simulink model "paralell_robot_D_2021"  (R2021a)
settings: Solver=VariableStepAuto  StartTime=0.0  StopTime=4*1.2  RelTol=1e-3
values from neighbouring files (symbols this model uses):
  B = 1.0    (= 1)    [paralell_robot_parameters.m]    (also in trajectory_generation.m = zeros(18,1))
  g = 9.81    [paralell_robot_parameters.m]    (also in robot_param.m)
  G = 0.8    [paralell_robot_parameters.m]
  I1_x = 50    [paralell_robot_parameters.m]    (also in robot_param.m)
  I1_y = 50    [paralell_robot_parameters.m]    (also in robot_param.m)
  I1_z = 50    [paralell_robot_parameters.m]    (also in robot_param.m)
  I2_x = 1    [paralell_robot_parameters.m]    (also in robot_param.m)
  I2_y = 20    [paralell_robot_parameters.m]    (also in robot_param.m)
  I2_z = 20    [paralell_robot_parameters.m]    (also in robot_param.m)
  I3_x = 0.5    [paralell_robot_parameters.m]    (also in robot_param.m)
  I3_y = 8    [paralell_robot_parameters.m]    (also in robot_param.m)
  I3_z = 8    [paralell_robot_parameters.m]    (also in robot_param.m)
  I4_x = 10    [paralell_robot_parameters.m]    (also in robot_param.m = 1)
  I4_y = 10    [paralell_robot_parameters.m]    (also in robot_param.m)
  I4_z = 10    [paralell_robot_parameters.m]    (also in robot_param.m)
  I5_x = 0.2    [paralell_robot_parameters.m]    (also in robot_param.m)
  I5_y = 1    [paralell_robot_parameters.m]    (also in robot_param.m)
  I5_z = 1    [paralell_robot_parameters.m]    (also in robot_param.m)
  I6_x = 2    [paralell_robot_parameters.m]    (also in robot_param.m)
  I6_y = 3    [paralell_robot_parameters.m]    (also in robot_param.m)
  I6_z = 2    [paralell_robot_parameters.m]    (also in robot_param.m)
  I7_x = 1    [paralell_robot_parameters.m]    (also in robot_param.m)
  I7_y = 18    [paralell_robot_parameters.m]    (also in robot_param.m)
  I7_z = 18    [paralell_robot_parameters.m]    (also in robot_param.m)
  I8_x = 0.5    [paralell_robot_parameters.m]    (also in robot_param.m = 0.2)
  I8_y = 2    [paralell_robot_parameters.m]    (also in robot_param.m)
  I8_z = 2    [paralell_robot_parameters.m]    (also in robot_param.m)
  I9_x = 1    [paralell_robot_parameters.m]    (also in robot_param.m)
  I9_y = 1    [paralell_robot_parameters.m]    (also in robot_param.m)
  I9_z = 1    [paralell_robot_parameters.m]    (also in robot_param.m)
  L1 = 0.240    (= 0.24)    [paralell_robot_parameters.m]    (also in robot_param.m)
  L2 = 0.800    (= 0.8)    [paralell_robot_parameters.m]    (also in robot_param.m)
  L3 = 1.050    (= 1.05)    [paralell_robot_parameters.m]    (also in robot_param.m)
  L4 = 1.175    [paralell_robot_parameters.m]    (also in robot_param.m)
  L5 = 0.225    [paralell_robot_parameters.m]    (also in robot_param.m)
  L6 = 0.200    (= 0.2)    [paralell_robot_parameters.m]    (also in robot_param.m)
  L7 = 0.235    [paralell_robot_parameters.m]    (also in robot_param.m)
  L8 = 0.248    [paralell_robot_parameters.m]    (also in robot_param.m)
  m1 = 750    [paralell_robot_parameters.m]    (also in robot_param.m)
  m2 = 250    [paralell_robot_parameters.m]    (also in robot_param.m)
  m3 = 150    [paralell_robot_parameters.m]    (also in robot_param.m)
  m4 = 500    [paralell_robot_parameters.m]    (also in robot_param.m)
  m5 = 50    [paralell_robot_parameters.m]    (also in robot_param.m = 150)
  m6 = 150    [paralell_robot_parameters.m]
  m7 = 200    [paralell_robot_parameters.m]    (also in robot_param.m)
  m8 = 100    [paralell_robot_parameters.m]    (also in robot_param.m)
  m9 = 50    [paralell_robot_parameters.m]    (also in robot_param.m)
  N = length(pt)-1    [trajectory_generation_quintic.m]
  PB = T+0.02    (= 0.12)    [paralell_robot_parameters.m]
  R = 0.0    (= 0)    [paralell_robot_parameters.m]
  T = 0.1    [paralell_robot_parameters.m]    (also in robot_param.m)
undefined symbols (not defined in the file or in its folder): A0, B0, B20, G0, g_ratioA, g_ratioH, g_ratioI, H0, I0, I_max, KdAt, KdAw, KdB2t, KdB2w, KdBt, KdBw, KdGt, KdGw, KdHt, KdHw, KiAt, KiAw, KiB2t, KiB2w, KiBt, KiBw, KiGt, KiGw, KiHt, KiHw, KmA, KmB, KmB2, KmG, KmH, KmI, KpAt, KpAw, KpB2t, KpB2w, KpBt, KpBw, KpGt, KpGw, KpHt, KpHw, KpIt, KpIw, X, Y, Z
libraries: sm_lib x152, nesl_utility x50, pid_lib x12
(part 1 of 5)
settings Model: Creator=tolla  LastModifiedBy=Bruker

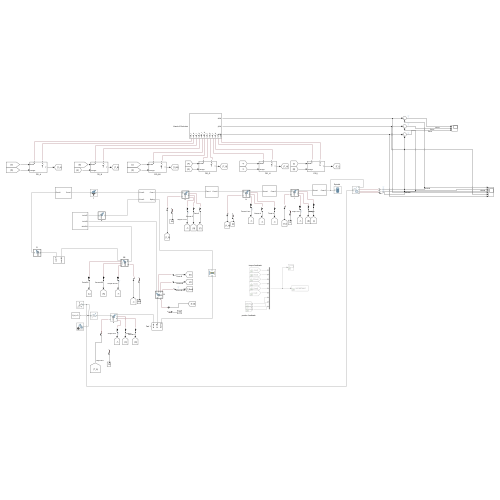
[thumbnail: Simulink's stored preview of the top-level diagram]
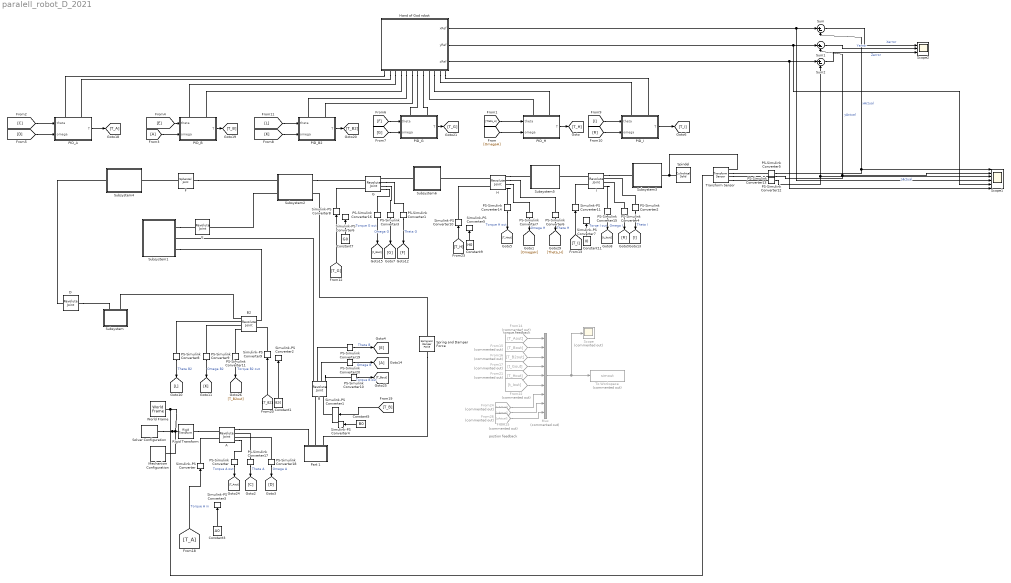
== system paralell_robot_D_2021 ==
  note: torque feedback
  note: postion feedback
  A : sm_lib/Joints/Revolute Joint  JointMode=Normal  SenseConstraintForce=off  SenseConstraintForceX=off  SenseConstraintForceY=off  SenseConstraintForceZ=off  SenseConstraintTorque=off  SenseConstraintTorqueX=off  SenseConstraintTorqueY=off  SenseConstraintTorqueZ=off  SenseTotalForce=off  SenseTotalForceX=off  SenseTotalForceY=off  SenseTotalForceZ=off  SenseTotalTorque=off  SenseTotalTorqueX=off  SenseTotalTorqueY=off  SenseTotalTorqueZ=off  CompositeWrenchDir=FollowerOnBase  CompositeWrenchFrame=BaseFrame  EquilibriumPosition=0  EquilibriumPositionUnits=deg  SpringStiffness=0  SpringStiffnessUnits=N*m/deg  DampingCoefficient=0  DampingCoefficientUnits=N*m/(deg/s)  TorqueActuationMode=InputTorque  MotionActuationMode=ComputedMotion  SensePosition=on  SenseVelocity=on  SenseAcceleration=off  SenseTorqueForce=on  SenseLowerLimitTorqueForce=off  SenseUpperLimitTorqueForce=off  LowerLimitSpecify=off  LowerLimitBound=-90  LowerLimitBoundUnits=deg  LowerLimitStiffness=1e4  LowerLimitStiffnessUnits=N*m/deg  LowerLimitDamping=10  LowerLimitDampingUnits=N*m/(deg/s)  LowerLimitTransitionRegionWidth=0.1  LowerLimitTransitionRegionWidthUnits=deg  UpperLimitSpecify=off  UpperLimitBound=90  UpperLimitBoundUnits=deg  UpperLimitStiffness=1e4  UpperLimitStiffnessUnits=N*m/deg  UpperLimitDamping=10  UpperLimitDampingUnits=N*m/(deg/s)  UpperLimitTransitionRegionWidth=0.1  UpperLimitTransitionRegionWidthUnits=deg  PositionTargetSpecify=on  PositionTargetPriority=High  PositionTargetValue=1.8800355033  PositionTargetValueUnits=rad  VelocityTargetSpecify=off  VelocityTargetPriority=High  VelocityTargetValue=0  VelocityTargetValueUnits=deg/s
  B : sm_lib/Joints/Revolute Joint  JointMode=Normal  SenseConstraintForce=off  SenseConstraintForceX=off  SenseConstraintForceY=off  SenseConstraintForceZ=off  SenseConstraintTorque=off  SenseConstraintTorqueX=off  SenseConstraintTorqueY=off  SenseConstraintTorqueZ=off  SenseTotalForce=off  SenseTotalForceX=off  SenseTotalForceY=off  SenseTotalForceZ=off  SenseTotalTorque=off  SenseTotalTorqueX=off  SenseTotalTorqueY=off  SenseTotalTorqueZ=off  CompositeWrenchDir=FollowerOnBase  CompositeWrenchFrame=BaseFrame  EquilibriumPosition=0  EquilibriumPositionUnits=deg  SpringStiffness=0  SpringStiffnessUnits=N*m/deg  DampingCoefficient=0  DampingCoefficientUnits=N*m/(deg/s)  TorqueActuationMode=InputTorque  MotionActuationMode=ComputedMotion  SensePosition=on  SenseVelocity=on  SenseAcceleration=off  SenseTorqueForce=on  SenseLowerLimitTorqueForce=off  SenseUpperLimitTorqueForce=off  LowerLimitSpecify=on  LowerLimitBound=-80  LowerLimitBoundUnits=deg  LowerLimitStiffness=1e4  LowerLimitStiffnessUnits=N*m/deg  LowerLimitDamping=10  LowerLimitDampingUnits=N*m/(deg/s)  LowerLimitTransitionRegionWidth=0.1  LowerLimitTransitionRegionWidthUnits=deg  UpperLimitSpecify=on  UpperLimitBound=80  UpperLimitBoundUnits=deg  UpperLimitStiffness=1e4  UpperLimitStiffnessUnits=N*m/deg  UpperLimitDamping=10  UpperLimitDampingUnits=N*m/(deg/s)  UpperLimitTransitionRegionWidth=0.1  UpperLimitTransitionRegionWidthUnits=deg  PositionTargetSpecify=on  PositionTargetPriority=High  PositionTargetValue=-0.198177592218  PositionTargetValueUnits=rad  VelocityTargetSpecify=off  VelocityTargetPriority=High  VelocityTargetValue=0  VelocityTargetValueUnits=deg/s
  B2 : sm_lib/Joints/Revolute Joint  JointMode=Normal  SenseConstraintForce=off  SenseConstraintForceX=off  SenseConstraintForceY=off  SenseConstraintForceZ=off  SenseConstraintTorque=off  SenseConstraintTorqueX=off  SenseConstraintTorqueY=off  SenseConstraintTorqueZ=off  SenseTotalForce=off  SenseTotalForceX=off  SenseTotalForceY=off  SenseTotalForceZ=off  SenseTotalTorque=off  SenseTotalTorqueX=off  SenseTotalTorqueY=off  SenseTotalTorqueZ=off  CompositeWrenchDir=FollowerOnBase  CompositeWrenchFrame=BaseFrame  EquilibriumPosition=0  EquilibriumPositionUnits=deg  SpringStiffness=0  SpringStiffnessUnits=N*m/deg  DampingCoefficient=0  DampingCoefficientUnits=N*m/(deg/s)  TorqueActuationMode=InputTorque  MotionActuationMode=ComputedMotion  SensePosition=on  SenseVelocity=on  SenseAcceleration=off  SenseTorqueForce=on  SenseLowerLimitTorqueForce=off  SenseUpperLimitTorqueForce=off  LowerLimitSpecify=off  LowerLimitBound=-90  LowerLimitBoundUnits=deg  LowerLimitStiffness=1e4  LowerLimitStiffnessUnits=N*m/deg  LowerLimitDamping=10  LowerLimitDampingUnits=N*m/(deg/s)  LowerLimitTransitionRegionWidth=0.1  LowerLimitTransitionRegionWidthUnits=deg  UpperLimitSpecify=off  UpperLimitBound=90  UpperLimitBoundUnits=deg  UpperLimitStiffness=1e4  UpperLimitStiffnessUnits=N*m/deg  UpperLimitDamping=10  UpperLimitDampingUnits=N*m/(deg/s)  UpperLimitTransitionRegionWidth=0.1  UpperLimitTransitionRegionWidthUnits=deg  PositionTargetSpecify=on  PositionTargetPriority=High  PositionTargetValue=0.024486078864  PositionTargetValueUnits=rad  VelocityTargetSpecify=off  VelocityTargetPriority=High  VelocityTargetValue=0  VelocityTargetValueUnits=deg/s
  Constant1 : Constant  Value=B20
  Constant11 : Constant  Value=I0
  Constant3 : Constant  Value=A0
  Constant5 : Constant  Value=B0
  Constant7 : Constant  Value=G0
  Constant9 : Constant  Value=H0
  D : sm_lib/Joints/Revolute Joint  JointMode=Normal  SenseConstraintForce=off  SenseConstraintForceX=off  SenseConstraintForceY=off  SenseConstraintForceZ=off  SenseConstraintTorque=off  SenseConstraintTorqueX=off  SenseConstraintTorqueY=off  SenseConstraintTorqueZ=off  SenseTotalForce=off  SenseTotalForceX=off  SenseTotalForceY=off  SenseTotalForceZ=off  SenseTotalTorque=off  SenseTotalTorqueX=off  SenseTotalTorqueY=off  SenseTotalTorqueZ=off  CompositeWrenchDir=FollowerOnBase  CompositeWrenchFrame=BaseFrame  EquilibriumPosition=0  EquilibriumPositionUnits=deg  SpringStiffness=0  SpringStiffnessUnits=N*m/deg  DampingCoefficient=0  DampingCoefficientUnits=N*m/(deg/s)  TorqueActuationMode=NoTorque  MotionActuationMode=ComputedMotion  SensePosition=off  SenseVelocity=off  SenseAcceleration=off  SenseTorqueForce=off  SenseLowerLimitTorqueForce=off  SenseUpperLimitTorqueForce=off  LowerLimitSpecify=off  LowerLimitBound=-90  LowerLimitBoundUnits=deg  LowerLimitStiffness=1e4  LowerLimitStiffnessUnits=N*m/deg  LowerLimitDamping=10  LowerLimitDampingUnits=N*m/(deg/s)  LowerLimitTransitionRegionWidth=0.1  LowerLimitTransitionRegionWidthUnits=deg  UpperLimitSpecify=off  UpperLimitBound=90  UpperLimitBoundUnits=deg  UpperLimitStiffness=1e4  UpperLimitStiffnessUnits=N*m/deg  UpperLimitDamping=10  UpperLimitDampingUnits=N*m/(deg/s)  UpperLimitTransitionRegionWidth=0.1  UpperLimitTransitionRegionWidthUnits=deg  PositionTargetSpecify=off  PositionTargetPriority=High  PositionTargetValue=-0.0059  PositionTargetValueUnits=rad  VelocityTargetSpecify=off  VelocityTargetPriority=High  VelocityTargetValue=0  VelocityTargetValueUnits=deg/s
  E : sm_lib/Joints/Revolute Joint  JointMode=Normal  SenseConstraintForce=off  SenseConstraintForceX=off  SenseConstraintForceY=off  SenseConstraintForceZ=off  SenseConstraintTorque=off  SenseConstraintTorqueX=off  SenseConstraintTorqueY=off  SenseConstraintTorqueZ=off  SenseTotalForce=off  SenseTotalForceX=off  SenseTotalForceY=off  SenseTotalForceZ=off  SenseTotalTorque=off  SenseTotalTorqueX=off  SenseTotalTorqueY=off  SenseTotalTorqueZ=off  CompositeWrenchDir=FollowerOnBase  CompositeWrenchFrame=BaseFrame  EquilibriumPosition=0  EquilibriumPositionUnits=deg  SpringStiffness=0  SpringStiffnessUnits=N*m/deg  DampingCoefficient=0  DampingCoefficientUnits=N*m/(deg/s)  TorqueActuationMode=NoTorque  MotionActuationMode=ComputedMotion  SensePosition=off  SenseVelocity=off  SenseAcceleration=off  SenseTorqueForce=off  SenseLowerLimitTorqueForce=off  SenseUpperLimitTorqueForce=off  LowerLimitSpecify=off  LowerLimitBound=-90  LowerLimitBoundUnits=deg  LowerLimitStiffness=1e4  LowerLimitStiffnessUnits=N*m/deg  LowerLimitDamping=10  LowerLimitDampingUnits=N*m/(deg/s)  LowerLimitTransitionRegionWidth=0.1  LowerLimitTransitionRegionWidthUnits=deg  UpperLimitSpecify=off  UpperLimitBound=90  UpperLimitBoundUnits=deg  UpperLimitStiffness=1e4  UpperLimitStiffnessUnits=N*m/deg  UpperLimitDamping=10  UpperLimitDampingUnits=N*m/(deg/s)  UpperLimitTransitionRegionWidth=0.1  UpperLimitTransitionRegionWidthUnits=deg  PositionTargetSpecify=off  PositionTargetPriority=High  PositionTargetValue=0.0059  PositionTargetValueUnits=rad  VelocityTargetSpecify=off  VelocityTargetPriority=High  VelocityTargetValue=0  VelocityTargetValueUnits=deg/s
  F : sm_lib/Joints/Spherical Joint  JointMode=Normal  SenseConstraintForce=off  SenseConstraintForceX=off  SenseConstraintForceY=off  SenseConstraintForceZ=off  SenseConstraintTorque=off  SenseConstraintTorqueX=off  SenseConstraintTorqueY=off  SenseConstraintTorqueZ=off  SenseTotalForce=off  SenseTotalForceX=off  SenseTotalForceY=off  SenseTotalForceZ=off  SenseTotalTorque=off  SenseTotalTorqueX=off  SenseTotalTorqueY=off  SenseTotalTorqueZ=off  CompositeWrenchDir=FollowerOnBase  CompositeWrenchFrame=BaseFrame  DefPosRotationMethod=None  DefPosRotationAngleUnits=deg  DefPosRotationStandardAxis=+Z  DefPosRotationAngle=0.0  DefPosRotationArbitraryAxis=[0 0 1]  DefPosFollAlignAxisA=+X  DefPosBaseAlignAxisA=+Y  DefPosFollAlignAxisB=+Y  DefPosBaseAlignAxisB=+Z  DefPosRotationSequenceAxes=FollowerAxes  DefPosRotationSequence=XYX  DefPosRotationSequenceAngles=[0 0 0]  DefPosRotationSequenceAnglesUnits=deg  DefPosRotationMatrix=[1 0 0; 0 1 0; 0 0 1]  EqPosRotationMethod=None  EqPosRotationAngleUnits=deg  EqPosRotationStandardAxis=+Z  EqPosRotationAngle=0.0  EqPosRotationArbitraryAxis=[0 0 1]  EqPosFollAlignAxisA=+X  EqPosBaseAlignAxisA=+Y  EqPosFollAlignAxisB=+Y  EqPosBaseAlignAxisB=+Z  EqPosRotationSequenceAxes=FollowerAxes  EqPosRotationSequence=XYX  EqPosRotationSequenceAngles=[0 0 0]  EqPosRotationSequenceAnglesUnits=deg  EqPosRotationMatrix=[1 0 0; 0 1 0; 0 0 1]  SpringStiffness=0  SpringStiffnessUnits=N*m/deg  DampingCoefficient=0  DampingCoefficientUnits=N*m/(deg/s)  ActuateTorqueX=off  ActuateTorqueY=off  ActuateTorqueZ=off  ActuateTorque=off  TorqueActuationMode=NoTorque  MotionActuationMode=ComputedMotion  ActuationFrame=BaseFrame  SensePosition=off  SenseVelocityX=off  SenseVelocityY=off  SenseVelocityZ=off  SenseVelocity=off  SenseAccelerationX=off  SenseAccelerationY=off  SenseAccelerationZ=off  SenseAcceleration=off  SenseTorqueX=off  SenseTorqueY=off  SenseTorqueZ=off  SenseTorqueForce=off  SenseLowerLimitTorqueMag=off  SenseUpperLimitTorqueMag=off  SensingFrame=BaseFrame  LowerLimitSpecify=off  LowerLimitBound=15  LowerLimitBoundUnits=deg  LowerLimitStiffness=1e4  LowerLimitStiffnessUnits=N*m/deg  LowerLimitDamping=10  LowerLimitDampingUnits=N*m/(deg/s)  LowerLimitTransitionRegionWidth=0.1  LowerLimitTransitionRegionWidthUnits=deg  UpperLimitSpecify=off  UpperLimitBound=45  UpperLimitBoundUnits=deg  UpperLimitStiffness=1e4  UpperLimitStiffnessUnits=N*m/deg  UpperLimitDamping=10  UpperLimitDampingUnits=N*m/(deg/s)  UpperLimitTransitionRegionWidth=0.1  UpperLimitTransitionRegionWidthUnits=deg  PositionTargetRotationMethod=None  PositionTargetRotationAngleUnits=deg  PositionTargetRotationStandardAxis=+Z  PositionTargetRotationAngle=0.0  PositionTargetRotationArbitraryAxis=[0 0 1]  PositionTargetFollAlignAxisA=+X  PositionTargetBaseAlignAxisA=+Y  PositionTargetFollAlignAxisB=+Y  PositionTargetBaseAlignAxisB=+Z  PositionTargetRotationSequenceAxes=FollowerAxes  PositionTargetRotationSequence=XYX  PositionTargetRotationSequenceAngles=[0 0 0]  PositionTargetRotationSequenceAnglesUnits=deg  PositionTargetRotationMatrix=[1 0 0; 0 1 0; 0 0 1]  PositionTargetSpecify=off  PositionTargetPriority=High  VelocityTargetValue=[0 0 0]  VelocityTargetValueUnits=deg/s  VelocityTargetSpecify=off  VelocityTargetPriority=High  VelocityTargetInFollowerFrame=on
  From14 : From  Commented=on  GotoTag=T_Aout
  From15 : From  Commented=on  GotoTag=T_Bout
  From16 : From  Commented=on  GotoTag=T_B2out
  From17 : From  Commented=on  GotoTag=t_Gout
  From21 : From  Commented=on  GotoTag=T_Hout
  From22 : From  Commented=on  GotoTag=t_Iout
  From24 : From  Commented=on  GotoTag=xActual
  From25 : From  Commented=on  GotoTag=yActual
  From26 : From  Commented=on  GotoTag=zActual
  G : sm_lib/Joints/Revolute Joint  JointMode=Normal  SenseConstraintForce=off  SenseConstraintForceX=off  SenseConstraintForceY=off  SenseConstraintForceZ=off  SenseConstraintTorque=off  SenseConstraintTorqueX=off  SenseConstraintTorqueY=off  SenseConstraintTorqueZ=off  SenseTotalForce=off  SenseTotalForceX=off  SenseTotalForceY=off  SenseTotalForceZ=off  SenseTotalTorque=off  SenseTotalTorqueX=off  SenseTotalTorqueY=off  SenseTotalTorqueZ=off  CompositeWrenchDir=FollowerOnBase  CompositeWrenchFrame=BaseFrame  EquilibriumPosition=0  EquilibriumPositionUnits=deg  SpringStiffness=0  SpringStiffnessUnits=N*m/deg  DampingCoefficient=0  DampingCoefficientUnits=N*m/(deg/s)  TorqueActuationMode=InputTorque  MotionActuationMode=ComputedMotion  SensePosition=on  SenseVelocity=on  SenseAcceleration=off  SenseTorqueForce=on  SenseLowerLimitTorqueForce=off  SenseUpperLimitTorqueForce=off  LowerLimitSpecify=off  LowerLimitBound=-90  LowerLimitBoundUnits=deg  LowerLimitStiffness=1e4  LowerLimitStiffnessUnits=N*m/deg  LowerLimitDamping=10  LowerLimitDampingUnits=N*m/(deg/s)  LowerLimitTransitionRegionWidth=0.1  LowerLimitTransitionRegionWidthUnits=deg  UpperLimitSpecify=off  UpperLimitBound=90  UpperLimitBoundUnits=deg  UpperLimitStiffness=1e4  UpperLimitStiffnessUnits=N*m/deg  UpperLimitDamping=10  UpperLimitDampingUnits=N*m/(deg/s)  UpperLimitTransitionRegionWidth=0.1  UpperLimitTransitionRegionWidthUnits=deg  PositionTargetSpecify=on  PositionTargetPriority=High  PositionTargetValue=-2.06664547582  PositionTargetValueUnits=rad  VelocityTargetSpecify=off  VelocityTargetPriority=High  VelocityTargetValue=0  VelocityTargetValueUnits=deg/s
  H : sm_lib/Joints/Revolute Joint  JointMode=Normal  SenseConstraintForce=off  SenseConstraintForceX=off  SenseConstraintForceY=off  SenseConstraintForceZ=off  SenseConstraintTorque=off  SenseConstraintTorqueX=off  SenseConstraintTorqueY=off  SenseConstraintTorqueZ=off  SenseTotalForce=off  SenseTotalForceX=off  SenseTotalForceY=off  SenseTotalForceZ=off  SenseTotalTorque=off  SenseTotalTorqueX=off  SenseTotalTorqueY=off  SenseTotalTorqueZ=off  CompositeWrenchDir=FollowerOnBase  CompositeWrenchFrame=BaseFrame  EquilibriumPosition=0  EquilibriumPositionUnits=deg  SpringStiffness=0  SpringStiffnessUnits=N*m/deg  DampingCoefficient=0  DampingCoefficientUnits=N*m/(deg/s)  TorqueActuationMode=InputTorque  MotionActuationMode=ComputedMotion  SensePosition=on  SenseVelocity=on  SenseAcceleration=off  SenseTorqueForce=on  SenseLowerLimitTorqueForce=off  SenseUpperLimitTorqueForce=off  LowerLimitSpecify=off  LowerLimitBound=-90  LowerLimitBoundUnits=deg  LowerLimitStiffness=1e4  LowerLimitStiffnessUnits=N*m/deg  LowerLimitDamping=10  LowerLimitDampingUnits=N*m/(deg/s)  LowerLimitTransitionRegionWidth=0.1  LowerLimitTransitionRegionWidthUnits=deg  UpperLimitSpecify=off  UpperLimitBound=90  UpperLimitBoundUnits=deg  UpperLimitStiffness=1e4  UpperLimitStiffnessUnits=N*m/deg  UpperLimitDamping=10  UpperLimitDampingUnits=N*m/(deg/s)  UpperLimitTransitionRegionWidth=0.1  UpperLimitTransitionRegionWidthUnits=deg  PositionTargetSpecify=on  PositionTargetPriority=High  PositionTargetValue=-0.3533098526406  PositionTargetValueUnits=rad  VelocityTargetSpecify=off  VelocityTargetPriority=High  VelocityTargetValue=0  VelocityTargetValueUnits=deg/s
  Hand of God robot : Subsystem
      settings: PortSchema="{\"entries\":[{\"content\":{\"sides\":[{\"content\":{\"connectorIds\":[]},\"type\":\"ConnectorPlacement.EquallySpacedRectSide\",\"uuid\":\"2da66bc7-d9c9-40f7-a607-c496d8ba411d\"},{\"content\":{\"connectorIds\":[\"RConn1\",\"RConn2\",\"RConn3\",\"RConn4\",\"RConn5\",\"RConn6\",\"RConn7\",\"RConn8\",\"RConn9\",\"RConn10\",\"RConn11\",\"RConn12\"],\"side\":\"RIGHT\"},\"type\":\"ConnectorPlacement.EquallySpacedRectSide\",\"uuid\":\"43301214-e3a9-4c79-a69b-8ea01f3b52fc\"},{\"content\":{\"connectorIds\":[],\"side\":\"TOP\"},\"type\":\"ConnectorPlacement.EquallySpacedRectSide\",\"uuid\":\"548f6eda-327e-49fc-954b-4c01b6ed85d8\"},{\"content\":{\"connectorIds\":[\"Out1\",\"Out2\",\"Out3\"],\"side\":\"BOTTOM\"},\"type\":\"ConnectorPlacement.EquallySpacedRectSide\",\"uuid\":\"9022aa30-dbbd-463e-a992-63fa47f152ea\"}]},\"type\":\"ConnectorPlacement.EquallySpacedConnector\",\"uuid\":\"1767b896-70e6-41af-96f0-a93ab9e9ba58\"}],\"packageUris\":[\"http://schema.mathworks.com/mf0/Connector/R2020b\"],\"version\":\"1.0\"}"
  I : sm_lib/Joints/Revolute Joint  JointMode=Normal  SenseConstraintForce=off  SenseConstraintForceX=off  SenseConstraintForceY=off  SenseConstraintForceZ=off  SenseConstraintTorque=off  SenseConstraintTorqueX=off  SenseConstraintTorqueY=off  SenseConstraintTorqueZ=off  SenseTotalForce=off  SenseTotalForceX=off  SenseTotalForceY=off  SenseTotalForceZ=off  SenseTotalTorque=off  SenseTotalTorqueX=off  SenseTotalTorqueY=off  SenseTotalTorqueZ=off  CompositeWrenchDir=FollowerOnBase  CompositeWrenchFrame=BaseFrame  EquilibriumPosition=0  EquilibriumPositionUnits=deg  SpringStiffness=0  SpringStiffnessUnits=N*m/deg  DampingCoefficient=0  DampingCoefficientUnits=N*m/(deg/s)  TorqueActuationMode=InputTorque  MotionActuationMode=ComputedMotion  SensePosition=on  SenseVelocity=on  SenseAcceleration=off  SenseTorqueForce=on  SenseLowerLimitTorqueForce=off  SenseUpperLimitTorqueForce=off  LowerLimitSpecify=off  LowerLimitBound=-90  LowerLimitBoundUnits=deg  LowerLimitStiffness=1e4  LowerLimitStiffnessUnits=N*m/deg  LowerLimitDamping=10  LowerLimitDampingUnits=N*m/(deg/s)  LowerLimitTransitionRegionWidth=0.1  LowerLimitTransitionRegionWidthUnits=deg  UpperLimitSpecify=off  UpperLimitBound=90  UpperLimitBoundUnits=deg  UpperLimitStiffness=1e4  UpperLimitStiffnessUnits=N*m/deg  UpperLimitDamping=10  UpperLimitDampingUnits=N*m/(deg/s)  UpperLimitTransitionRegionWidth=0.1  UpperLimitTransitionRegionWidthUnits=deg  PositionTargetSpecify=on  PositionTargetPriority=High  PositionTargetValue=-2.0937842723459  PositionTargetValueUnits=rad  VelocityTargetSpecify=off  VelocityTargetPriority=High  VelocityTargetValue=0  VelocityTargetValueUnits=deg/s
  Mechanism Configuration : sm_lib/Utilities/Mechanism Configuration  UniformGravity=Constant  GravityVector=[0 0 -g]  GravityUnits=m/s^2  LinearizationDelta=0.001  JointModeTransitionNonlinearIterations=2
  Mux : Mux  Commented=on  Inputs=9
  PID_A : Subsystem
      settings: PortSchema="{\"entries\":[{\"content\":{\"sides\":[{\"content\":{\"connectorIds\":[\"In1\",\"In2\"]},\"type\":\"ConnectorPlacement.EquallySpacedRectSide\",\"uuid\":\"88fb2923-d567-49e7-965d-54b8b92ddc6d\"},{\"content\":{\"connectorIds\":[\"Out1\"],\"side\":\"RIGHT\"},\"type\":\"ConnectorPlacement.EquallySpacedRectSide\",\"uuid\":\"46ea93fe-e994-4ece-a41c-2bcb9003d689\"},{\"content\":{\"connectorIds\":[\"LConn1\",\"LConn2\"],\"side\":\"TOP\"},\"type\":\"ConnectorPlacement.EquallySpacedRectSide\",\"uuid\":\"eb03c7d4-9431-42de-84d2-d91d69b85d14\"}]},\"type\":\"ConnectorPlacement.EquallySpacedConnector\",\"uuid\":\"bf201109-a610-49f1-9baa-d8b74c8b6eeb\"}],\"packageUris\":[\"http://schema.mathworks.com/mf0/Connector/R2020b\"],\"version\":\"1.0\"}"
  PID_B : Subsystem
      settings: PortSchema="{\"entries\":[{\"content\":{\"sides\":[{\"content\":{\"connectorIds\":[\"In1\",\"In2\"]},\"type\":\"ConnectorPlacement.EquallySpacedRectSide\",\"uuid\":\"88fb2923-d567-49e7-965d-54b8b92ddc6d\"},{\"content\":{\"connectorIds\":[\"Out1\"],\"side\":\"RIGHT\"},\"type\":\"ConnectorPlacement.EquallySpacedRectSide\",\"uuid\":\"46ea93fe-e994-4ece-a41c-2bcb9003d689\"},{\"content\":{\"connectorIds\":[\"LConn1\",\"LConn2\"],\"side\":\"TOP\"},\"type\":\"ConnectorPlacement.EquallySpacedRectSide\",\"uuid\":\"eb03c7d4-9431-42de-84d2-d91d69b85d14\"}]},\"type\":\"ConnectorPlacement.EquallySpacedConnector\",\"uuid\":\"bf201109-a610-49f1-9baa-d8b74c8b6eeb\"}],\"packageUris\":[\"http://schema.mathworks.com/mf0/Connector/R2020b\"],\"version\":\"1.0\"}"
  PID_B2 : Subsystem
      settings: PortSchema="{\"entries\":[{\"content\":{\"sides\":[{\"content\":{\"connectorIds\":[\"In1\",\"In2\"]},\"type\":\"ConnectorPlacement.EquallySpacedRectSide\",\"uuid\":\"88fb2923-d567-49e7-965d-54b8b92ddc6d\"},{\"content\":{\"connectorIds\":[\"Out1\"],\"side\":\"RIGHT\"},\"type\":\"ConnectorPlacement.EquallySpacedRectSide\",\"uuid\":\"46ea93fe-e994-4ece-a41c-2bcb9003d689\"},{\"content\":{\"connectorIds\":[\"LConn1\",\"LConn2\"],\"side\":\"TOP\"},\"type\":\"ConnectorPlacement.EquallySpacedRectSide\",\"uuid\":\"eb03c7d4-9431-42de-84d2-d91d69b85d14\"}]},\"type\":\"ConnectorPlacement.EquallySpacedConnector\",\"uuid\":\"bf201109-a610-49f1-9baa-d8b74c8b6eeb\"}],\"packageUris\":[\"http://schema.mathworks.com/mf0/Connector/R2020b\"],\"version\":\"1.0\"}"
  PID_G : Subsystem
      settings: PortSchema="{\"entries\":[{\"content\":{\"sides\":[{\"content\":{\"connectorIds\":[\"In1\",\"In2\"]},\"type\":\"ConnectorPlacement.EquallySpacedRectSide\",\"uuid\":\"88fb2923-d567-49e7-965d-54b8b92ddc6d\"},{\"content\":{\"connectorIds\":[\"Out1\"],\"side\":\"RIGHT\"},\"type\":\"ConnectorPlacement.EquallySpacedRectSide\",\"uuid\":\"46ea93fe-e994-4ece-a41c-2bcb9003d689\"},{\"content\":{\"connectorIds\":[\"LConn1\",\"LConn2\"],\"side\":\"TOP\"},\"type\":\"ConnectorPlacement.EquallySpacedRectSide\",\"uuid\":\"eb03c7d4-9431-42de-84d2-d91d69b85d14\"}]},\"type\":\"ConnectorPlacement.EquallySpacedConnector\",\"uuid\":\"bf201109-a610-49f1-9baa-d8b74c8b6eeb\"}],\"packageUris\":[\"http://schema.mathworks.com/mf0/Connector/R2020b\"],\"version\":\"1.0\"}"
  PID_H : Subsystem
      settings: PortSchema="{\"entries\":[{\"content\":{\"sides\":[{\"content\":{\"connectorIds\":[\"In1\",\"In2\"]},\"type\":\"ConnectorPlacement.EquallySpacedRectSide\",\"uuid\":\"88fb2923-d567-49e7-965d-54b8b92ddc6d\"},{\"content\":{\"connectorIds\":[\"Out1\"],\"side\":\"RIGHT\"},\"type\":\"ConnectorPlacement.EquallySpacedRectSide\",\"uuid\":\"46ea93fe-e994-4ece-a41c-2bcb9003d689\"},{\"content\":{\"connectorIds\":[\"LConn1\",\"LConn2\"],\"side\":\"TOP\"},\"type\":\"ConnectorPlacement.EquallySpacedRectSide\",\"uuid\":\"eb03c7d4-9431-42de-84d2-d91d69b85d14\"}]},\"type\":\"ConnectorPlacement.EquallySpacedConnector\",\"uuid\":\"bf201109-a610-49f1-9baa-d8b74c8b6eeb\"}],\"packageUris\":[\"http://schema.mathworks.com/mf0/Connector/R2020b\"],\"version\":\"1.0\"}"
  PID_I : Subsystem
      settings: PortSchema="{\"entries\":[{\"content\":{\"sides\":[{\"content\":{\"connectorIds\":[\"In1\",\"In2\"]},\"type\":\"ConnectorPlacement.EquallySpacedRectSide\",\"uuid\":\"88fb2923-d567-49e7-965d-54b8b92ddc6d\"},{\"content\":{\"connectorIds\":[\"Out1\"],\"side\":\"RIGHT\"},\"type\":\"ConnectorPlacement.EquallySpacedRectSide\",\"uuid\":\"46ea93fe-e994-4ece-a41c-2bcb9003d689\"},{\"content\":{\"connectorIds\":[\"LConn1\",\"LConn2\"],\"side\":\"TOP\"},\"type\":\"ConnectorPlacement.EquallySpacedRectSide\",\"uuid\":\"eb03c7d4-9431-42de-84d2-d91d69b85d14\"}]},\"type\":\"ConnectorPlacement.EquallySpacedConnector\",\"uuid\":\"bf201109-a610-49f1-9baa-d8b74c8b6eeb\"}],\"packageUris\":[\"http://schema.mathworks.com/mf0/Connector/R2020b\"],\"version\":\"1.0\"}"
  PS-Simulink Converter{,5,10..16} (9 alike) : nesl_utility/PS-Simulink Converter  PhysicalDomain=network_engine_domain  SubClassName=ps_output  LeftPortType=input  RightPortType=output  PseudoPeriodic=off  Frequencies=[]  VectorFormat=inherit  Unit=inherit  AffineConversion=off
      settings: SourceProductBaseCode=SS,PW,VE
  PS-Simulink Converter{1..4,6..9,17..20} (12 alike) : nesl_utility/PS-Simulink Converter  PhysicalDomain=network_engine_domain  SubClassName=ps_output  LeftPortType=input  RightPortType=output  PseudoPeriodic=off  Frequencies=[]  VectorFormat=1-D array  Unit=inherit  AffineConversion=off
      settings: SourceProductBaseCode=SS,PW,VE
  Part 1 : Subsystem
  Rigid Transform : sm_lib/Frames and Transforms/Rigid Transform  TranslationMethod=Cartesian  TranslationStandardOffset=0  TranslationLengthUnit=m  TranslationStandardAxis=+Z  TranslationCartesianOffset=[0 0 0]  TranslationROffset=0  TranslationROffsetUnits=m  TranslationZOffset=0  TranslationZOffsetUnits=m  TranslationThetaOffset=0  TranslationThetaOffsetUnits=deg  RotationMethod=None  RotationAngleUnits=deg  RotationStandardAxis=+Z  RotationAngle=0.0  RotationArbitraryAxis=[0 0 1]  FollAlignAxisA=+X  BaseAlignAxisA=+Y  FollAlignAxisB=+Y  BaseAlignAxisB=+Z  RotationSequenceAxes=FollowerAxes  RotationSequence=XYX  RotationSequenceAngles=[0 0 0]  RotationSequenceAnglesUnits=deg  RotationMatrix=[1 0 0; 0 1 0; 0 0 1]
  Scope : Scope  Commented=on
  Scope1 : Scope  NumInputPorts=6
  Scope2 : Scope  NumInputPorts=3
  Simulink-PS Converter{,8..11} (5 alike) : nesl_utility/Simulink-PS Converter  PhysicalDomain=network_engine_domain  SubClassName=ps_input  LeftPortType=input  RightPortType=output  PseudoPeriodic=off  Frequencies=[]  NoiseDistribution=none  NoiseParameters=[]  Unit=1  AffineConversion=off  FilteringAndDerivatives=provide  SimscapeFilterOrder=1  InputFilterTimeConstant=0.001  UdotUserProvided=0
      settings: SourceProductBaseCode=SS,PW,VE
  Simulink-PS Converter1 : nesl_utility/Simulink-PS Converter  PhysicalDomain=network_engine_domain  SubClassName=ps_input  LeftPortType=input  RightPortType=output  PseudoPeriodic=off  Frequencies=[]  NoiseDistribution=none  NoiseParameters=[]  Unit=1  AffineConversion=off  FilteringAndDerivatives=provide  SimscapeFilterOrder=2  InputFilterTimeConstant=0.001  UdotUserProvided=0
      settings: SourceProductBaseCode=SS,PW,VE
  Simulink-PS Converter{2..7} (6 alike) : nesl_utility/Simulink-PS Converter  PhysicalDomain=network_engine_domain  SubClassName=ps_input  LeftPortType=input  RightPortType=output  PseudoPeriodic=off  Frequencies=[]  NoiseDistribution=none  NoiseParameters=[]  Unit=1  AffineConversion=off  FilteringAndDerivatives=filter  SimscapeFilterOrder=2  InputFilterTimeConstant=0.001  UdotUserProvided=0
      settings: SourceProductBaseCode=SS,PW,VE
  Solver Configuration : nesl_utility/Solver Configuration  PhysicalDomain=network_engine_domain  SubClassName=solver  LeftPortType=input  RightPortType=generic  Tones=[]  Harmonics=[]  SimulateNoise=off  Profile=off  UseLocalSampling=off  EnableSwitchedLinearOptims=on  FrequencyDomain=off  UseCCode=off  RelTol=0.001  AbsTol=1e-06  MinStep=1e-09  ToWorkspace=off  RevertToSquareIcSolve=off  NumHomotopyIterations=100  PhasorMode=off  PhasorModeNumHarmonics=1  IndexReductionMethod=DerivativeReplacement  DoDC=off  ResidualTolerance=1e-09  UseLocalSolver=off  LocalSolverChoice=NE_BACKWARD_EULER_ADVANCER  LocalSolverSampleTime=0.001  DoFixedCost=off  MaxNonlinIter=3  MaxModeIter=2  ComputeImpulses=off  ImpulseIterations=2  LinearAlgebra=auto  LinearAlgebraNumThread=0  EquationFormulation=NE_TIME_EF  DelaysMemoryBudget=1024  AutomaticFiltering=on  FilteringTimeConstant=0.001  PartitionStorageMethod=AS_NEEDED  PartitionMemoryBudget=1024  PartitionMethod=ROBUST
      settings: SourceProductBaseCode=SS,PW,VE
  Spindel : sm_lib/Body Elements/Cylindrical Solid  GraphicAmbientColor=[0.15 0.15 0.15 1.0]  BasedOnType=Density  CenterOfMass=[0 0 0]  CenterOfMassUnits=m  GraphicDiffuseColor=[0.0 0.0 0.0]  CylinderLength=0.03  CylinderLengthUnits=m  CylinderRadius=0.01  CylinderRadiusUnits=m  Density=1000  DensityUnits=kg/m^3  DoExposeReferenceFrame=on  GraphicEmissiveColor=[0.0 0.0 0.0 1.0]  ExportEntireGeometry=off  SerializedFrames=<Frames/>  MarkerShape=Sphere  MarkerSize=10  GraphicType=FromGeometry  InertiaType=PointMass  Mass=1  MassUnits=kg  MomentsOfInertia=[1 1 1]  MomentsOfInertiaUnits=kg*m^2  GraphicOpacity=1.0  ProductsOfInertia=[0 0 0]  ProductsOfInertiaUnits=kg*m^2  GraphicShininess=75  GraphicSpecularColor=[0.5 0.5 0.5 1.0]  GraphicVisPropType=SimpleVisualProperties
  Spring and Damper Force : sm_lib/Forces and Torques/Spring and Damper Force  NaturalLength=0.75  NaturalLengthUnits=m  SpringStiffness=120000  SpringStiffnessUnits=N/m  DampingCoefficient=0  DampingCoefficientUnits=N/(m/s)  SenseForce=off
  Subsystem : Subsystem
  Subsystem1 : Subsystem
  Subsystem2 : Subsystem
  Subsystem3 : Subsystem
  Subsystem4 : Subsystem
  Subsystem5 : Subsystem
  Subsystem6 : Subsystem
  Sum : Sum  Inputs=|+-
  Sum1 : Sum  Inputs=|+-
  Sum2 : Sum  Inputs=|+-
  To Workspace : ToWorkspace  Commented=on  VariableName=simout  SaveFormat=Timeseries  SampleTime=-1
  Transform Sensor : sm_lib/Frames and Transforms/Transform Sensor  MeasurementFrame=World  SenseAngle=off  SenseAxis=off  SenseAngle1=off  SenseAngle2=off  SenseAngle3=off  SenseQ=off  SenseR=off  SenseOmegaX=off  SenseOmegaY=off  SenseOmegaZ=off  SenseOmega1=off  SenseOmega2=off  SenseOmega3=off  SenseQDot=off  SenseRDot=off  SenseAlphaX=off  SenseAlphaY=off  SenseAlphaZ=off  SenseAlpha1=off  SenseAlpha2=off  SenseAlpha3=off  SenseQDDot=off  SenseRDDot=off  SenseX=on  SenseY=on  SenseZ=on  SenseRad=off  SenseAzim=off  SenseDist=off  SenseInc=off  SenseXDot=off  SenseYDot=off  SenseZDot=off  SenseRadDot=off  SenseAzimDot=off  SenseDistDot=off  SenseIncDot=off  SenseXDDot=off  SenseYDDot=off  SenseZDDot=off  SenseRadDDot=off  SenseAzimDDot=off  SenseDistDDot=off  SenseIncDDot=off
  World Frame : sm_lib/Frames and Transforms/World Frame
  wires:
  [D] -> PID_A/2(omega)
  [C] -> PID_A/1(theta)
  [E] -> PID_B/1(theta)
  [A] -> PID_B/2(omega)
  PID_B/1(T) -> [T_B]
  [L] -> PID_B2/1(theta)
  PID_B2/1(T) -> [T_B2]
  [I] -> PID_I/1(theta)
  PID_I/1(T) -> [T_I]
  PID_H/1(T) -> [T_H]
  [F] -> PID_G/1(theta)
  PID_G/1(T) -> [T_G]
  PS-Simulink Converter19/1 -> [E]  "Theta B"
  PS-Simulink Converter17/1 -> [C]  "Theta A"
  PS-Simulink Converter18/1 -> [D]  "Omega A"
  PS-Simulink Converter20/1 -> [A]  "Omega B"
  PS-Simulink Converter10/1 -> [T_Bout]  "Torque B out"
  PS-Simulink Converter9/1 -> [K]  "Omega B2"
  PS-Simulink Converter8/1 -> [L]  "Theta B2"
  PS-Simulink Converter/1 -> [T_Aout]  "Torque A out"
  PS-Simulink Converter7/1 -> [OmegaH]  "Omega H"
  PS-Simulink Converter11/1 -> [T_B2out]  "Torque B2 out"
  PS-Simulink Converter1/1 -> [F]  "Theta G"
  PS-Simulink Converter2/1 -> [I]  "Theta I"
  [Theta_H] -> PID_H/1(theta)
  PS-Simulink Converter3/1 -> [G]  "Omega G"
  PS-Simulink Converter4/1 -> [R]  "Omega I"
  PS-Simulink Converter6/1 -> [Theta_H]  "Theta H"
  PS-Simulink Converter5/1 -> Sum/2, Scope1/1  "xActual"
  PS-Simulink Converter12/1 -> Sum1/2, Scope1/2  "yActual"
  PS-Simulink Converter13/1 -> Sum2/2, Scope1/3  "zActual"
  PS-Simulink Converter14/1 -> [T_Hout]  "Torque H out"
  PS-Simulink Converter15/1 -> [t_Iout]  "Torqe I out"
  PS-Simulink Converter16/1 -> [t_Gout]  "Torque G out"
  Mux/1 -> Scope/1, To Workspace/1
  From14/1 -> Mux/1
  From15/1 -> Mux/2
  From16/1 -> Mux/3
  From17/1 -> Mux/4
  From21/1 -> Mux/5
  From22/1 -> Mux/6
  From24/1 -> Mux/7
  From25/1 -> Mux/8
  From26/1 -> Mux/9
  Hand of God robot/1(xRef) -> Scope1/4, Sum/1
  Hand of God robot/2(yRef) -> Scope1/5, Sum1/1
  Hand of God robot/3(zRef) -> Scope1/6, Sum2/1
  Sum/1 -> Scope2/1  "Xerror"
  Sum1/1 -> Scope2/2  "Yerror"
  Sum2/1 -> Scope2/3  "Zerror"
  PID_A/1(T) -> [T_A]
  [K] -> PID_B2/2(omega)
  [G] -> PID_G/2(omega)
  [OmegaH] -> PID_H/2(omega)
  [R] -> PID_I/2(omega)
  [T_G] -> Simulink-PS Converter8/1
  Constant7/1 -> Simulink-PS Converter6/1
  [T_A] -> Simulink-PS Converter/1  "Torque A in"
  Constant3/1 -> Simulink-PS Converter3/1
  [T_B] -> Simulink-PS Converter1/1
  Constant5/1 -> Simulink-PS Converter4/1
  Constant1/1 -> Simulink-PS Converter2/1
  [T_B2] -> Simulink-PS Converter9/1
  Constant9/1 -> Simulink-PS Converter5/1
  [T_H] -> Simulink-PS Converter10/1
  Constant11/1 -> Simulink-PS Converter7/1
  [T_I] -> Simulink-PS Converter11/1
  connections:
  Hand of God robot/RConn1 -- PID_A/LConn1
  Hand of God robot/RConn3 -- PID_B/LConn1
  Hand of God robot/RConn5 -- PID_B2/LConn1
  Hand of God robot/RConn11 -- PID_I/LConn1
  PID_H/LConn1 -- Hand of God robot/RConn9
  Solver Configuration/RConn1 -- Transform Sensor/LConn1 -- World Frame/RConn1 -- Mechanism Configuration/RConn1 -- Rigid Transform/LConn1
  Spring and Damper Force/LConn1 -- Part 1/LConn3
  Subsystem4/LConn1 -- D/RConn1
  B/RConn1 -- Subsystem1/RConn2
  PS-Simulink Converter17/LConn1 -- A/RConn2
  Part 1/LConn2 -- B/LConn1
  Subsystem1/RConn3 -- B2/LConn1
  PS-Simulink Converter18/LConn1 -- A/RConn3
  A/RConn1 -- Part 1/LConn1
  B2/RConn1 -- Subsystem/RConn2
  B/RConn4 -- PS-Simulink Converter10/LConn1
  D/LConn1 -- Subsystem/RConn1
  B2/RConn4 -- PS-Simulink Converter11/LConn1
  PS-Simulink Converter19/LConn1 -- B/RConn2
  H/RConn2 -- PS-Simulink Converter6/LConn1
  H/RConn3 -- PS-Simulink Converter7/LConn1
  F/LConn1 -- Subsystem4/RConn1
  PS-Simulink Converter20/LConn1 -- B/RConn3
  Rigid Transform/RConn1 -- A/LConn1
  A/RConn4 -- PS-Simulink Converter/LConn1
  Subsystem1/RConn1 -- E/LConn1
  B2/RConn2 -- PS-Simulink Converter8/LConn1
  B2/RConn3 -- PS-Simulink Converter9/LConn1
  PS-Simulink Converter2/LConn1 -- I/RConn2
  I/RConn1 -- Subsystem3/LConn1
  Spindel/RConn1 -- Transform Sensor/RConn1 -- Subsystem3/RConn1
  H/RConn1 -- Subsystem5/LConn1
  I/LConn1 -- Subsystem5/RConn1
  H/LConn1 -- Subsystem6/RConn1
  Subsystem6/LConn1 -- G/RConn1
  Subsystem2/RConn1 -- G/LConn1
  F/RConn1 -- Subsystem2/LConn1
  Subsystem2/LConn2 -- E/RConn1
  Spring and Damper Force/RConn1 -- Subsystem2/RConn2
  G/RConn2 -- PS-Simulink Converter1/LConn1
  G/RConn3 -- PS-Simulink Converter3/LConn1
  PS-Simulink Converter4/LConn1 -- I/RConn3
  Transform Sensor/RConn2 -- PS-Simulink Converter5/LConn1
  Transform Sensor/RConn3 -- PS-Simulink Converter12/LConn1
  Transform Sensor/RConn4 -- PS-Simulink Converter13/LConn1
  H/RConn4 -- PS-Simulink Converter14/LConn1
  I/RConn4 -- PS-Simulink Converter15/LConn1
  G/RConn4 -- PS-Simulink Converter16/LConn1
  Hand of God robot/RConn7 -- PID_G/LConn1
  Hand of God robot/RConn2 -- PID_A/LConn2
  Hand of God robot/RConn4 -- PID_B/LConn2
  Hand of God robot/RConn6 -- PID_B2/LConn2
  Hand of God robot/RConn8 -- PID_G/LConn2
  Hand of God robot/RConn10 -- PID_H/LConn2
  Hand of God robot/RConn12 -- PID_I/LConn2
  Simulink-PS Converter11/RConn1 -- I/LConn2
  Simulink-PS Converter10/RConn1 -- H/LConn2
  Simulink-PS Converter8/RConn1 -- G/LConn2
  Simulink-PS Converter9/RConn1 -- B2/LConn2
  Simulink-PS Converter/RConn1 -- A/LConn2
  Simulink-PS Converter1/RConn1 -- B/LConn2
